simulink model "SF105A_MotCurrRegVltgLimr"  (R2013b)
settings: Solver=FixedStepDiscrete  SolverMode=SingleTasking  StartTime=0.0  StopTime=1  FixedStep=0.00025  RelTol=1e-3
undefined symbols (not defined in the file): ARCHGLBPRM_2OVERSQRT3_ULS_F32, ARCHGLBPRM_2PI_ULS_F32, BRDGVLTGHILIM_VOLT_F32, ELECGLBPRM_PWMPERDNOMX2_SEC_F32, F32TOU16OVR2PI_ULS_F32, MotCurrRegCfgCurrLoopSecOrderTrfFctEna, MotCurrRegCfgMotRVirtDax, MotCurrRegCfgMotRVirtQax, MotCurrRegVltgLimrCurrLoaScarSlewRate, MotCurrRegVltgLimrDaxAntiWdupCoeff, MotCurrRegVltgLimrDualEcuLoaScarSlewRate, MotCurrRegVltgLimrIvtrLoaScarSlewRate, MotCurrRegVltgLimrMotCurrPredEna, MotCurrRegVltgLimrMotCurrPredTi, MotCurrRegVltgLimrMotCurrQaxRefMdfnRplEna, MotCurrRegVltgLimrMotVltgBrdgFilEna, MotCurrRegVltgLimrMotVltgDaxIntglHiLim, MotCurrRegVltgLimrMotVltgDaxIntglLoLim, MotCurrRegVltgLimrMotVltgQaxFfFilEna, MotCurrRegVltgLimrMotVltgQaxIntglHiLim, MotCurrRegVltgLimrMotVltgQaxIntglLoLim, MotCurrRegVltgLimrQaxAntiWdupCoeff, MotCurrRegVltgLimrQaxAntiWdupScagDi, MotRefMdlFbCtrlDi, MotRefMdlIvtrDeadTiBrdgVltgSca, SysSt1, ZERO_VOLT_F32
libraries: NxtrLim x15, Fil x4, simulink x3, NxtrMax x2, NxtrMin x2
(part 3 of 5)

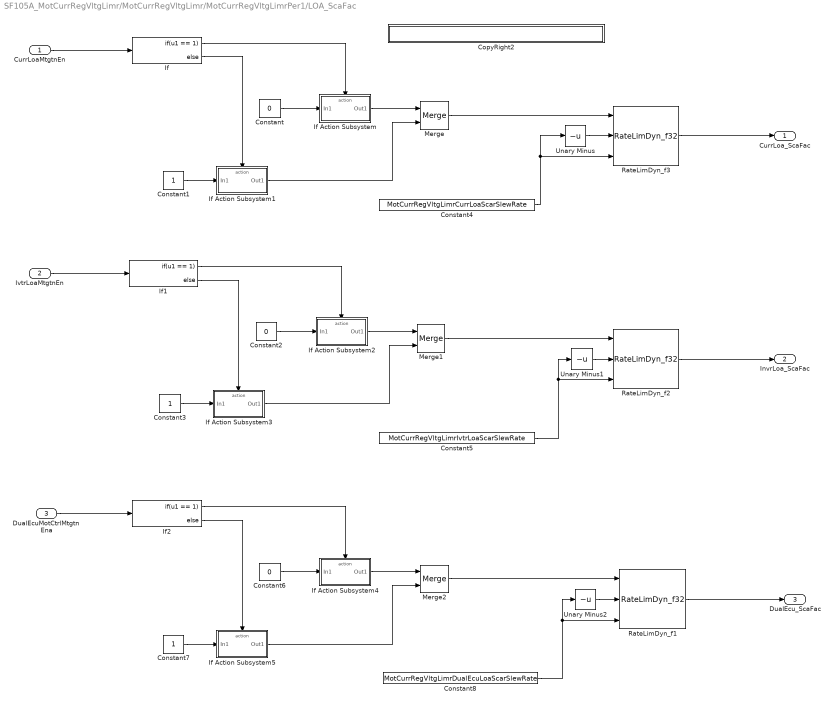
== system SF105A_MotCurrRegVltgLimr/MotCurrRegVltgLimr/MotCurrRegVltgLimrPer1/LOA_ScaFac ==
  CurrLoaMtgtnEn : Inport  RequirementInfo={'linktype_rmi_doors' '0000bb44 (/E-STEER Core/SubSystem Specifications/Application Functions/SF99/SF105A Current Regulator and Voltage Limiter)' '#SF105A_102' 'true' 'REQ: SF105A_102' '' } %GIDa_74016de8_2d3d_4e44_85d8_d4113689b030
  IvtrLoaMtgtnEn : Inport  RequirementInfo={'linktype_rmi_doors' '0000bb44 (/E-STEER Core/SubSystem Specifications/Application Functions/SF99/SF105A Current Regulator and Voltage Limiter)' '#SF105A_156' 'true' 'REQ: SF105A_156' '' } %GIDa_6f58899e_8eab_433e_baee_2993c9bd34be  Port=2
  DualEcuMotCtrlMtgtnEna : Inport  RequirementInfo={'linktype_rmi_doors' '0000bb44 (/E-STEER Core/SubSystem Specifications/Application Functions/SF99/SF105A Current Regulator and Voltage Limiter)' '#SF105A_156' 'true' 'REQ: SF105A_156' '' ; 'linktype_rmi_doors' '0000bb44 (/E-STEER Core/SubSystem Specifications/Application Functions/SF99/SF105A Current Regulator and Voltage Limiter)' '#SF105A_214' 'true' 'REQ: SF105A_214' '' } %GIDa_736db6b8_8a98_4c01_a4db_8969b61e8301  Port=3
  Constant : Constant  RequirementInfo={'linktype_rmi_doors' '0000bb44 (/E-STEER Core/SubSystem Specifications/Application Functions/SF99/SF105A Current Regulator and Voltage Limiter)' '#SF105A_102' 'true' 'REQ: SF105A_102' '' } %GIDa_9e5edeaa_9753_4523_84fc_d0edb0466ebb  Value=0  OutDataTypeStr=single
  Constant1 : Constant  RequirementInfo={'linktype_rmi_doors' '0000bb44 (/E-STEER Core/SubSystem Specifications/Application Functions/SF99/SF105A Current Regulator and Voltage Limiter)' '#SF105A_102' 'true' 'REQ: SF105A_102' '' } %GIDa_414e47fe_925f_4ace_960c_c6b1b25b4ef2  OutDataTypeStr=single
  Constant2 : Constant  RequirementInfo={'linktype_rmi_doors' '0000bb44 (/E-STEER Core/SubSystem Specifications/Application Functions/SF99/SF105A Current Regulator and Voltage Limiter)' '#SF105A_156' 'true' 'REQ: SF105A_156' '' } %GIDa_1b7b7f87_2781_4c0b_92e7_3da3ba5adda7  Value=0  OutDataTypeStr=single
  Constant3 : Constant  RequirementInfo={'linktype_rmi_doors' '0000bb44 (/E-STEER Core/SubSystem Specifications/Application Functions/SF99/SF105A Current Regulator and Voltage Limiter)' '#SF105A_156' 'true' 'REQ: SF105A_156' '' } %GIDa_009e418e_db5b_41d9_ae78_f46b7f47c2f9  OutDataTypeStr=single
  Constant4 : Constant  RequirementInfo={'linktype_rmi_doors' '0000bb44 (/E-STEER Core/SubSystem Specifications/Application Functions/SF99/SF105A Current Regulator and Voltage Limiter)' '#SF105A_101' 'true' 'REQ: SF105A_101' '' } %GIDa_4127ceec_6765_4e92_b839_f1bde89d8c0b  Value=MotCurrRegVltgLimrCurrLoaScarSlewRate
  Constant5 : Constant  RequirementInfo={'linktype_rmi_doors' '0000bb44 (/E-STEER Core/SubSystem Specifications/Application Functions/SF99/SF105A Current Regulator and Voltage Limiter)' '#SF105A_158' 'true' 'REQ: SF105A_158' '' } %GIDa_d375279a_c0b4_445f_88b4_097dc89d2371  Value=MotCurrRegVltgLimrIvtrLoaScarSlewRate
  Constant6 : Constant  RequirementInfo={'linktype_rmi_doors' '0000bb44 (/E-STEER Core/SubSystem Specifications/Application Functions/SF99/SF105A Current Regulator and Voltage Limiter)' '#SF105A_156' 'true' 'REQ: SF105A_156' '' ; 'linktype_rmi_doors' '0000bb44 (/E-STEER Core/SubSystem Specifications/Application Functions/SF99/SF105A Current Regulator and Voltage Limiter)' '#SF105A_214' 'true' 'REQ: SF105A_214' '' } %GIDa_1132c686_87fe_415f_a0bc_4e5d655024ab  Value=0  OutDataTypeStr=single
  Constant7 : Constant  RequirementInfo={'linktype_rmi_doors' '0000bb44 (/E-STEER Core/SubSystem Specifications/Application Functions/SF99/SF105A Current Regulator and Voltage Limiter)' '#SF105A_156' 'true' 'REQ: SF105A_156' '' ; 'linktype_rmi_doors' '0000bb44 (/E-STEER Core/SubSystem Specifications/Application Functions/SF99/SF105A Current Regulator and Voltage Limiter)' '#SF105A_214' 'true' 'REQ: SF105A_214' '' } %GIDa_7ef12da6_ad43_483e_a835_c5dd150fe6fe  OutDataTypeStr=single
  Constant8 : Constant  RequirementInfo={'linktype_rmi_doors' '0000bb44 (/E-STEER Core/SubSystem Specifications/Application Functions/SF99/SF105A Current Regulator and Voltage Limiter)' '#SF105A_213' 'true' 'REQ: SF105A_213' '' } %GIDa_fc42a242_7564_4710_9c19_eef5c8ae2cee  Value=MotCurrRegVltgLimrDualEcuLoaScarSlewRate
  CopyRight2 : Subsystem  Description=|  mask(Copyright Information){none=on}
      | Copyright info block.                                               
      |                                                                     
      | Place copyright information at the top of every subsystem in design.
      mask prompts: none "No parameters"
      mask help: Place copyright information at the top of every subsystem in design.
      mask Display:
      | NxtrConf = 'Nexteer Confidential';
      | 
      | sys = bdroot; %handle for the current model ("system")
      | first = get_param(sys,'Created');
      | if(isempty(first))
      |     first = datestr(now,'yyyy');
      | else
      |     first = first(end-3:end);  %year is last four digits
      | end
      | 
      | last = get_param(sys,'LastModifiedDate');
      | if isempty(last)
      |     last = datestr(now,'yyyy');
      | else
      |     last = last(end-3:end);
      | end
      | 
      | if strcmp(first,last)
      |     fprintf('%s -- Copyright %s Nexteer',NxtrConf,first)
      | else
      |     fprintf('%s -- %s%s- %s Nexteer',NxtrConf,char(169),first,last)
      | end
  If : If  RequirementInfo={'linktype_rmi_doors' '0000bb44 (/E-STEER Core/SubSystem Specifications/Application Functions/SF99/SF105A Current Regulator and Voltage Limiter)' '#SF105A_102' 'true' 'REQ: SF105A_102' '' } %GIDa_3a91bae6_7fe9_4df3_8189_f002690391f2  IfExpression=u1 == 1
  If Action Subsystem : Subsystem  RequirementInfo={'linktype_rmi_doors' '0000bb44 (/E-STEER Core/SubSystem Specifications/Application Functions/SF99/SF105A Current Regulator and Voltage Limiter)' '#SF105A_102' 'true' 'REQ: SF105A_102' '' } %GIDa_4746905c_4450_4de8_aeb6_d31492493c35  TreatAsAtomicUnit=on
  If Action Subsystem1 : Subsystem  RequirementInfo={'linktype_rmi_doors' '0000bb44 (/E-STEER Core/SubSystem Specifications/Application Functions/SF99/SF105A Current Regulator and Voltage Limiter)' '#SF105A_102' 'true' 'REQ: SF105A_102' '' } %GIDa_3824dd5c_a3c5_4e02_bf52_4a1d9300439b  TreatAsAtomicUnit=on
  If Action Subsystem2 : Subsystem  RequirementInfo={'linktype_rmi_doors' '0000bb44 (/E-STEER Core/SubSystem Specifications/Application Functions/SF99/SF105A Current Regulator and Voltage Limiter)' '#SF105A_156' 'true' 'REQ: SF105A_156' '' } %GIDa_1af216f2_cb25_4b77_bb8c_abc2dc18253e  TreatAsAtomicUnit=on
  If Action Subsystem3 : Subsystem  RequirementInfo={'linktype_rmi_doors' '0000bb44 (/E-STEER Core/SubSystem Specifications/Application Functions/SF99/SF105A Current Regulator and Voltage Limiter)' '#SF105A_156' 'true' 'REQ: SF105A_156' '' } %GIDa_f1b7b46f_b59a_420d_a525_ef233d17b094  TreatAsAtomicUnit=on
  If Action Subsystem4 : Subsystem  RequirementInfo={'linktype_rmi_doors' '0000bb44 (/E-STEER Core/SubSystem Specifications/Application Functions/SF99/SF105A Current Regulator and Voltage Limiter)' '#SF105A_156' 'true' 'REQ: SF105A_156' '' ; 'linktype_rmi_doors' '0000bb44 (/E-STEER Core/SubSystem Specifications/Application Functions/SF99/SF105A Current Regulator and Voltage Limiter)' '#SF105A_214' 'true' 'REQ: SF105A_214' '' } %GIDa_6d2e553f_9dcf_4646_b57e_342b22099bc6  TreatAsAtomicUnit=on
  If Action Subsystem5 : Subsystem  RequirementInfo={'linktype_rmi_doors' '0000bb44 (/E-STEER Core/SubSystem Specifications/Application Functions/SF99/SF105A Current Regulator and Voltage Limiter)' '#SF105A_156' 'true' 'REQ: SF105A_156' '' ; 'linktype_rmi_doors' '0000bb44 (/E-STEER Core/SubSystem Specifications/Application Functions/SF99/SF105A Current Regulator and Voltage Limiter)' '#SF105A_214' 'true' 'REQ: SF105A_214' '' } %GIDa_45a5a307_dfa1_464a_845e_5937a4578355  TreatAsAtomicUnit=on
  If1 : If  RequirementInfo={'linktype_rmi_doors' '0000bb44 (/E-STEER Core/SubSystem Specifications/Application Functions/SF99/SF105A Current Regulator and Voltage Limiter)' '#SF105A_156' 'true' 'REQ: SF105A_156' '' } %GIDa_08038fbf_a660_4706_ace0_908cef9a7a3c  IfExpression=u1 == 1
  If2 : If  RequirementInfo={'linktype_rmi_doors' '0000bb44 (/E-STEER Core/SubSystem Specifications/Application Functions/SF99/SF105A Current Regulator and Voltage Limiter)' '#SF105A_156' 'true' 'REQ: SF105A_156' '' ; 'linktype_rmi_doors' '0000bb44 (/E-STEER Core/SubSystem Specifications/Application Functions/SF99/SF105A Current Regulator and Voltage Limiter)' '#SF105A_214' 'true' 'REQ: SF105A_214' '' } %GIDa_d47c7b75_0445_4629_a8f6_7d3cc89f6b1e  IfExpression=u1 == 1
  Merge : Merge  RequirementInfo={'linktype_rmi_doors' '0000bb44 (/E-STEER Core/SubSystem Specifications/Application Functions/SF99/SF105A Current Regulator and Voltage Limiter)' '#SF105A_102' 'true' 'REQ: SF105A_102' '' } %GIDa_02e5c2a5_d864_4ef7_8f58_89b7f0e83ac4
  Merge1 : Merge  RequirementInfo={'linktype_rmi_doors' '0000bb44 (/E-STEER Core/SubSystem Specifications/Application Functions/SF99/SF105A Current Regulator and Voltage Limiter)' '#SF105A_156' 'true' 'REQ: SF105A_156' '' } %GIDa_1411ac7b_0602_4079_91ff_3bf75b7f8933
  Merge2 : Merge  RequirementInfo={'linktype_rmi_doors' '0000bb44 (/E-STEER Core/SubSystem Specifications/Application Functions/SF99/SF105A Current Regulator and Voltage Limiter)' '#SF105A_156' 'true' 'REQ: SF105A_156' '' ; 'linktype_rmi_doors' '0000bb44 (/E-STEER Core/SubSystem Specifications/Application Functions/SF99/SF105A Current Regulator and Voltage Limiter)' '#SF105A_214' 'true' 'REQ: SF105A_214' '' } %GIDa_b21e043f_9e48_4dac_a088_0ae5e3077f20
  RateLimDyn_f1 : NxtrLim/RateLimDyn_f32  RequirementInfo={'linktype_rmi_doors' '0000bb44 (/E-STEER Core/SubSystem Specifications/Application Functions/SF99/SF105A Current Regulator and Voltage Limiter)' '#SF105A_215' 'true' 'REQ: SF105A_215' '' } %GIDa_febcb8d3_d490_462d_9585_cc90d4e1d855  StVar=DualEcuLoaScarPrev  Ts=ELECGLBPRM_PWMPERDNOMX2_SEC_F32
      settings: AttributesFormatString=StVar: %<StVar>
  RateLimDyn_f2 : NxtrLim/RateLimDyn_f32  StVar=IvtrLoaScarPrev  Ts=ELECGLBPRM_PWMPERDNOMX2_SEC_F32
      settings: AttributesFormatString=StVar: %<StVar>
  RateLimDyn_f3 : NxtrLim/RateLimDyn_f32  StVar=CurrLoaScarPrev  Ts=ELECGLBPRM_PWMPERDNOMX2_SEC_F32
      settings: AttributesFormatString=StVar: %<StVar>
  Unary Minus : UnaryMinus  RequirementInfo={'linktype_rmi_doors' '0000bb44 (/E-STEER Core/SubSystem Specifications/Application Functions/SF99/SF105A Current Regulator and Voltage Limiter)' '#SF105A_101' 'true' 'REQ: SF105A_101' '' } %GIDa_2742d1db_4c29_4c43_bc00_21ac76a60273
  Unary Minus1 : UnaryMinus  RequirementInfo={'linktype_rmi_doors' '0000bb44 (/E-STEER Core/SubSystem Specifications/Application Functions/SF99/SF105A Current Regulator and Voltage Limiter)' '#SF105A_158' 'true' 'REQ: SF105A_158' '' } %GIDa_35918956_e63f_4f48_ad3b_713daa2d1a68
  Unary Minus2 : UnaryMinus  RequirementInfo={'linktype_rmi_doors' '0000bb44 (/E-STEER Core/SubSystem Specifications/Application Functions/SF99/SF105A Current Regulator and Voltage Limiter)' '#SF105A_158' 'true' 'REQ: SF105A_158' '' } %GIDa_c3ad0f7f_3bfe_4cdc_ba65_f783df0f12a2
  CurrLoa_ScaFac : Outport  RequirementInfo={'linktype_rmi_doors' '0000bb44 (/E-STEER Core/SubSystem Specifications/Application Functions/SF99/SF105A Current Regulator and Voltage Limiter)' '#SF105A_102' 'true' 'REQ: SF105A_102' '' } %GIDa_45fecacb_2175_43de_a689_6a1c7683416a
  InvrLoa_ScaFac : Outport  RequirementInfo={'linktype_rmi_doors' '0000bb44 (/E-STEER Core/SubSystem Specifications/Application Functions/SF99/SF105A Current Regulator and Voltage Limiter)' '#SF105A_156' 'true' 'REQ: SF105A_156' '' } %GIDa_392678cc_9a17_4a2c_ba15_6492b437acac  Port=2
  DualEcu_ScaFac : Outport  RequirementInfo={'linktype_rmi_doors' '0000bb44 (/E-STEER Core/SubSystem Specifications/Application Functions/SF99/SF105A Current Regulator and Voltage Limiter)' '#SF105A_156' 'true' 'REQ: SF105A_156' '' } %GIDa_aaab24fd_64b0_48fa_9ed0_c4d4e741348c  Port=3
  wires:
  RateLimDyn_f3/1 -> CurrLoa_ScaFac/1
  RateLimDyn_f2/1 -> InvrLoa_ScaFac/1
  CurrLoaMtgtnEn/1 -> If/1
  If/1 -> If Action Subsystem/Action
  If/2 -> If Action Subsystem1/Action
  If Action Subsystem/1(Out1) -> Merge/1
  If Action Subsystem1/1(Out1) -> Merge/2
  Merge/1 -> RateLimDyn_f3/1
  Constant/1 -> If Action Subsystem/1(In1)
  Constant1/1 -> If Action Subsystem1/1(In1)
  If1/1 -> If Action Subsystem2/Action
  If1/2 -> If Action Subsystem3/Action
  If Action Subsystem2/1(Out1) -> Merge1/1
  If Action Subsystem3/1(Out1) -> Merge1/2
  Constant2/1 -> If Action Subsystem2/1(In1)
  Constant3/1 -> If Action Subsystem3/1(In1)
  Merge1/1 -> RateLimDyn_f2/1
  IvtrLoaMtgtnEn/1 -> If1/1
  Unary Minus/1 -> RateLimDyn_f3/2
  Constant4/1 -> RateLimDyn_f3/3, Unary Minus/1
  Constant5/1 -> RateLimDyn_f2/3, Unary Minus1/1
  Unary Minus1/1 -> RateLimDyn_f2/2
  RateLimDyn_f1/1 -> DualEcu_ScaFac/1
  If2/1 -> If Action Subsystem4/Action
  If2/2 -> If Action Subsystem5/Action
  If Action Subsystem4/1(Out1) -> Merge2/1
  If Action Subsystem5/1(Out1) -> Merge2/2
  Constant6/1 -> If Action Subsystem4/1(In1)
  Constant7/1 -> If Action Subsystem5/1(In1)
  Merge2/1 -> RateLimDyn_f1/1
  DualEcuMotCtrlMtgtnEna/1 -> If2/1
  Constant8/1 -> RateLimDyn_f1/3, Unary Minus2/1
  Unary Minus2/1 -> RateLimDyn_f1/2

== system SF105A_MotCurrRegVltgLimr/MotCurrRegVltgLimr/MotCurrRegVltgLimrPer1/MotCurr_ErrCalc_Dax ==
  MotCurr_DaxCmd : Inport  RequirementInfo={'linktype_rmi_doors' '0000bb44 (/E-STEER Core/SubSystem Specifications/Application Functions/SF99/SF105A Current Regulator and Voltage Limiter)' '#SF105A_79' 'true' 'REQ: SF105A_79' '' } %GIDa_9f860954_e875_4c8d_8e1d_5693f49ff45b
  MotCurr_DaxCmd_Max : Inport  RequirementInfo={'linktype_rmi_doors' '0000bb44 (/E-STEER Core/SubSystem Specifications/Application Functions/SF99/SF105A Current Regulator and Voltage Limiter)' '#SF105A_79' 'true' 'REQ: SF105A_79' '' } %GIDa_059e93a2_947a_47bb_8dd6_2243dd2f4f72  Port=2
  MotCurrModif_Dax : Inport  RequirementInfo={'linktype_rmi_doors' '0000bb44 (/E-STEER Core/SubSystem Specifications/Application Functions/SF99/SF105A Current Regulator and Voltage Limiter)' '#SF105A_80' 'true' 'REQ: SF105A_80' '' } %GIDa_0a5f56fa_a877_4df4_9019_19b65ccf742b  Port=3
  AntiWdup_CmdScag_Dax : Inport  RequirementInfo={'linktype_rmi_doors' '0000bb44 (/E-STEER Core/SubSystem Specifications/Application Functions/SF99/SF105A Current Regulator and Voltage Limiter)' '#SF105A_79' 'true' 'REQ: SF105A_79' '' } %GIDa_16448b7e_ab4b_4b1d_9cde_07b89661d2d9  Port=4
  Add : Sum  RequirementInfo={'linktype_rmi_doors' '0000bb44 (/E-STEER Core/SubSystem Specifications/Application Functions/SF99/SF105A Current Regulator and Voltage Limiter)' '#SF105A_79' 'true' 'REQ: SF105A_79' '' } %GIDa_39dd1027_d310_4f71_96a2_2a266e8bfe38  Inputs=-+
  Add1 : Sum  RequirementInfo={'linktype_rmi_doors' '0000bb44 (/E-STEER Core/SubSystem Specifications/Application Functions/SF99/SF105A Current Regulator and Voltage Limiter)' '#SF105A_79' 'true' 'REQ: SF105A_79' '' ; 'linktype_rmi_doors' '0000bb44 (/E-STEER Core/SubSystem Specifications/Application Functions/SF99/SF105A Current Regulator and Voltage Limiter)' '#SF105A_80' 'true' 'REQ: SF105A_80' '' } %GIDa_29048c9a_b932_4a00_8976_f9e9609904a4
  Add2 : Sum  RequirementInfo={'linktype_rmi_doors' '0000bb44 (/E-STEER Core/SubSystem Specifications/Application Functions/SF99/SF105A Current Regulator and Voltage Limiter)' '#SF105A_80' 'true' 'REQ: SF105A_80' '' } %GIDa_390b17ed_9d59_44c9_82bb_54ff4b90a4f8  Inputs=+-
  Constant : Constant  RequirementInfo={'linktype_rmi_doors' '0000bb44 (/E-STEER Core/SubSystem Specifications/Application Functions/SF99/SF105A Current Regulator and Voltage Limiter)' '#SF105A_79' 'true' 'REQ: SF105A_79' '' } %GIDa_71ff8474_cc08_4c6f_98c7_9495352e7f22  OutDataTypeStr=single
  CopyRight2 : Subsystem  Description=|  mask(Copyright Information){none=on}
      | Copyright info block.                                               
      |                                                                     
      | Place copyright information at the top of every subsystem in design.
      mask prompts: none "No parameters"
      mask help: Place copyright information at the top of every subsystem in design.
      mask Display:
      | NxtrConf = 'Nexteer Confidential';
      | 
      | sys = bdroot; %handle for the current model ("system")
      | first = get_param(sys,'Created');
      | if(isempty(first))
      |     first = datestr(now,'yyyy');
      | else
      |     first = first(end-3:end);  %year is last four digits
      | end
      | 
      | last = get_param(sys,'LastModifiedDate');
      | if isempty(last)
      |     last = datestr(now,'yyyy');
      | else
      |     last = last(end-3:end);
      | end
      | 
      | if strcmp(first,last)
      |     fprintf('%s -- Copyright %s Nexteer',NxtrConf,first)
      | else
      |     fprintf('%s -- %s%s- %s Nexteer',NxtrConf,char(169),first,last)
      | end
  Data Store Write : DataStoreWrite  DataStoreName=dMotCurrRegVltgLimrMotCurrCmdScaDax
  Data Store Write1 : DataStoreWrite  DataStoreName=dMotCurrRegVltgLimrMotCurrCmdErrDax
  LimStat_f32 : NxtrLim/LimStat_f32  RequirementInfo={'linktype_rmi_doors' '0000bb44 (/E-STEER Core/SubSystem Specifications/Application Functions/SF99/SF105A Current Regulator and Voltage Limiter)' '#SF105A_194' 'true' 'REQ: SF105A_194' '' } %GIDa_41824742_1c4e_4aae_9c40_6d1680dffacc  LoLim=0  HiLim=MOTCURRHILIM_AMPR_F32
      settings: AttributesFormatString=|
      | Low Limit: %<LoLim>
      | High Limit:%<HiLim>
  Product : Product  RequirementInfo={'linktype_rmi_doors' '0000bb44 (/E-STEER Core/SubSystem Specifications/Application Functions/SF99/SF105A Current Regulator and Voltage Limiter)' '#SF105A_79' 'true' 'REQ: SF105A_79' '' } %GIDa_865b35e4_9b9d_4019_bb82_f747255cb73b
  Product1 : Product  RequirementInfo={'linktype_rmi_doors' '0000bb44 (/E-STEER Core/SubSystem Specifications/Application Functions/SF99/SF105A Current Regulator and Voltage Limiter)' '#SF105A_79' 'true' 'REQ: SF105A_79' '' } %GIDa_d60d7378_f447_4ef8_b073_e1658ac34c86
  CmdErr_Dax : Outport  RequirementInfo={'linktype_rmi_doors' '0000bb44 (/E-STEER Core/SubSystem Specifications/Application Functions/SF99/SF105A Current Regulator and Voltage Limiter)' '#SF105A_80' 'true' 'REQ: SF105A_80' '' } %GIDa_fb394d4d_5f75_43b4_b8c6_8763df3a229d
  wires:
  MotCurr_DaxCmd/1 -> Product/1
  AntiWdup_CmdScag_Dax/1 -> Product/2, Add/1
  Constant/1 -> Add/2
  Add/1 -> Product1/1
  MotCurr_DaxCmd_Max/1 -> Product1/2
  Product1/1 -> Add1/2
  Product/1 -> Add1/1
  Add1/1 -> LimStat_f32/1
  Add2/1 -> Data Store Write1/1, CmdErr_Dax/1
  MotCurrModif_Dax/1 -> Add2/2
  LimStat_f32/1 -> Add2/1, Data Store Write/1

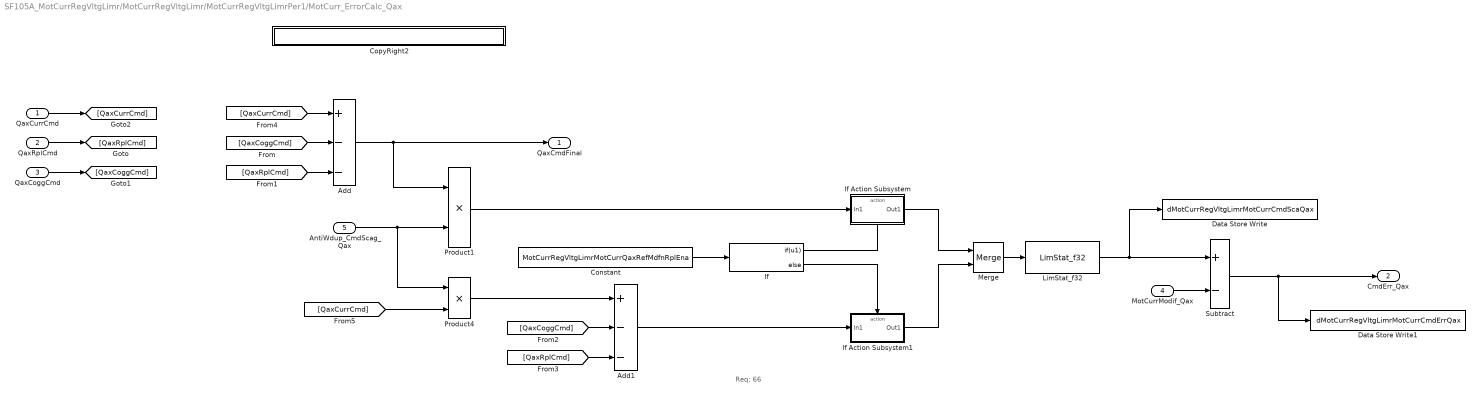
== system SF105A_MotCurrRegVltgLimr/MotCurrRegVltgLimr/MotCurrRegVltgLimrPer1/MotCurr_ErrorCalc_Qax ==
  note: Req: 66
  QaxCurrCmd : Inport
  QaxRplCmd : Inport  Port=2
  QaxCoggCmd : Inport  Port=3
  MotCurrModif_Qax : Inport  RequirementInfo={'linktype_rmi_doors' '0000bb44 (/E-STEER Core/SubSystem Specifications/Application Functions/SF99/SF105A Current Regulator and Voltage Limiter)' '#SF105A_68' 'true' 'REQ: SF105A_68' '' } %GIDa_7ddb042c_949f_40bd_a5a0_caaccdad8aec  Port=4
  AntiWdup_CmdScag_Qax : Inport  RequirementInfo={'linktype_rmi_doors' '0000bb44 (/E-STEER Core/SubSystem Specifications/Application Functions/SF99/SF105A Current Regulator and Voltage Limiter)' '#SF105A_66' 'true' 'REQ: SF105A_66' '' } %GIDa_f11ef98d_60e0_4a29_bcf5_371694c4b8ce  Port=5
  Add : Sum  RequirementInfo={'linktype_rmi_doors' '0000bb44 (/E-STEER Core/SubSystem Specifications/Application Functions/SF99/SF105A Current Regulator and Voltage Limiter)' '#SF105A_67' 'true' 'REQ: SF105A_67' '' } %GIDa_824a2f17_525f_4037_bf25_6f84ed62cd1c  Inputs=+--
  Add1 : Sum  RequirementInfo={'linktype_rmi_doors' '0000bb44 (/E-STEER Core/SubSystem Specifications/Application Functions/SF99/SF105A Current Regulator and Voltage Limiter)' '#SF105A_67' 'true' 'REQ: SF105A_67' '' ; 'linktype_rmi_doors' '0000bb44 (/E-STEER Core/SubSystem Specifications/Application Functions/SF99/SF105A Current Regulator and Voltage Limiter)' '#SF105A_68' 'true' 'REQ: SF105A_68' '' ; 'linktype_rmi_doors' '0000bb44 (/E-STEER Core/SubSystem Specifications/Application Functions/SF99/SF105A Current Regulator and Voltage Limiter)' '#SF105A_66' 'true' 'REQ: SF105A_66' '' } %GIDa_68034fa4_dd2b_4432_96f4_ee6556315ecf  Inputs=+--
  Constant : Constant  RequirementInfo={'linktype_rmi_doors' '0000bb44 (/E-STEER Core/SubSystem Specifications/Application Functions/SF99/SF105A Current Regulator and Voltage Limiter)' '#SF105A_66' 'true' 'REQ: SF105A_66' '' } %GIDa_9ec7087e_f41f_4423_86a7_6e625803caeb  Value=MotCurrRegVltgLimrMotCurrQaxRefMdfnRplEna
  CopyRight2 : Subsystem  Description=|  mask(Copyright Information){none=on}
      | Copyright info block.                                               
      |                                                                     
      | Place copyright information at the top of every subsystem in design.
      mask prompts: none "No parameters"
      mask help: Place copyright information at the top of every subsystem in design.
      mask Display:
      | NxtrConf = 'Nexteer Confidential';
      | 
      | sys = bdroot; %handle for the current model ("system")
      | first = get_param(sys,'Created');
      | if(isempty(first))
      |     first = datestr(now,'yyyy');
      | else
      |     first = first(end-3:end);  %year is last four digits
      | end
      | 
      | last = get_param(sys,'LastModifiedDate');
      | if isempty(last)
      |     last = datestr(now,'yyyy');
      | else
      |     last = last(end-3:end);
      | end
      | 
      | if strcmp(first,last)
      |     fprintf('%s -- Copyright %s Nexteer',NxtrConf,first)
      | else
      |     fprintf('%s -- %s%s- %s Nexteer',NxtrConf,char(169),first,last)
      | end
  Data Store Write : DataStoreWrite  DataStoreName=dMotCurrRegVltgLimrMotCurrCmdScaQax
  Data Store Write1 : DataStoreWrite  DataStoreName=dMotCurrRegVltgLimrMotCurrCmdErrQax
  If : If  RequirementInfo={'linktype_rmi_doors' '0000bb44 (/E-STEER Core/SubSystem Specifications/Application Functions/SF99/SF105A Current Regulator and Voltage Limiter)' '#SF105A_66' 'true' 'REQ: SF105A_66' '' } %GIDa_3422f6ba_ed31_4d28_a209_ee709dd11907  IfExpression=u1
  If Action Subsystem : Subsystem  RequirementInfo={'linktype_rmi_doors' '0000bb44 (/E-STEER Core/SubSystem Specifications/Application Functions/SF99/SF105A Current Regulator and Voltage Limiter)' '#SF105A_66' 'true' 'REQ: SF105A_66' '' } %GIDa_cff3645e_70eb_479a_8cd2_a8659d70b1bb  TreatAsAtomicUnit=on
  If Action Subsystem1 : Subsystem  RequirementInfo={'linktype_rmi_doors' '0000bb44 (/E-STEER Core/SubSystem Specifications/Application Functions/SF99/SF105A Current Regulator and Voltage Limiter)' '#SF105A_66' 'true' 'REQ: SF105A_66' '' } %GIDa_5c53fa27_9bd9_46be_8574_f721519fc2a6  TreatAsAtomicUnit=on
  LimStat_f32 : NxtrLim/LimStat_f32  RequirementInfo={'linktype_rmi_doors' '0000bb44 (/E-STEER Core/SubSystem Specifications/Application Functions/SF99/SF105A Current Regulator and Voltage Limiter)' '#SF105A_192' 'true' 'REQ: SF105A_192' '' } %GIDa_31cf29ce_c2ae_4e26_a267_244a0aa9250f  LoLim=MOTCURRLOLIM_AMPR_F32  HiLim=MOTCURRHILIM_AMPR_F32
      settings: AttributesFormatString=|
      | Low Limit: %<LoLim>
      | High Limit:%<HiLim>
  Merge : Merge  RequirementInfo={'linktype_rmi_doors' '0000bb44 (/E-STEER Core/SubSystem Specifications/Application Functions/SF99/SF105A Current Regulator and Voltage Limiter)' '#SF105A_66' 'true' 'REQ: SF105A_66' '' } %GIDa_0142320b_7588_4c2a_92e0_9d1571f759a1
  Product1 : Product  RequirementInfo={'linktype_rmi_doors' '0000bb44 (/E-STEER Core/SubSystem Specifications/Application Functions/SF99/SF105A Current Regulator and Voltage Limiter)' '#SF105A_66' 'true' 'REQ: SF105A_66' '' } %GIDa_00046f93_3b3c_43ee_b28c_8f0dba5d6301
  Product4 : Product  RequirementInfo={'linktype_rmi_doors' '0000bb44 (/E-STEER Core/SubSystem Specifications/Application Functions/SF99/SF105A Current Regulator and Voltage Limiter)' '#SF105A_66' 'true' 'REQ: SF105A_66' '' ; 'linktype_rmi_doors' '0000bb44 (/E-STEER Core/SubSystem Specifications/Application Functions/SF99/SF105A Current Regulator and Voltage Limiter)' '#SF105A_67' 'true' 'REQ: SF105A_67' '' ; 'linktype_rmi_doors' '0000bb44 (/E-STEER Core/SubSystem Specifications/Application Functions/SF99/SF105A Current Regulator and Voltage Limiter)' '#SF105A_66' 'true' 'REQ: SF105A_66' '' } %GIDa_5eda651c_d9cf_4592_83a1_ad2c6ced6304
  Subtract : Sum  RequirementInfo={'linktype_rmi_doors' '0000bb44 (/E-STEER Core/SubSystem Specifications/Application Functions/SF99/SF105A Current Regulator and Voltage Limiter)' '#SF105A_68' 'true' 'REQ: SF105A_68' '' } %GIDa_847c6db2_b488_4579_a9b0_6b38d1c11d10  Inputs=+-
  QaxCmdFinal : Outport
  CmdErr_Qax : Outport  RequirementInfo={'linktype_rmi_doors' '0000bb44 (/E-STEER Core/SubSystem Specifications/Application Functions/SF99/SF105A Current Regulator and Voltage Limiter)' '#SF105A_68' 'true' 'REQ: SF105A_68' '' } %GIDa_89496b6d_771a_4c11_b3f5_27b7e28477ad  Port=2
  wires:
  [QaxCurrCmd] -> Product4/2
  MotCurrModif_Qax/1 -> Subtract/2
  Subtract/1 -> Data Store Write1/1, CmdErr_Qax/1
  Product4/1 -> Add1/1
  Add1/1 -> If Action Subsystem1/1(In1)
  QaxRplCmd/1 -> [QaxRplCmd]
  QaxCoggCmd/1 -> [QaxCoggCmd]
  [QaxCoggCmd] -> Add/2
  [QaxRplCmd] -> Add/3
  [QaxCoggCmd] -> Add1/2
  [QaxRplCmd] -> Add1/3
  QaxCurrCmd/1 -> [QaxCurrCmd]
  [QaxCurrCmd] -> Add/1
  AntiWdup_CmdScag_Qax/1 -> Product4/1, Product1/2
  Add/1 -> Product1/1, QaxCmdFinal/1
  Product1/1 -> If Action Subsystem/1(In1)
  Constant/1 -> If/1
  If/1 -> If Action Subsystem/Action
  If/2 -> If Action Subsystem1/Action
  If Action Subsystem1/1(Out1) -> Merge/2
  If Action Subsystem/1(Out1) -> Merge/1
  Merge/1 -> LimStat_f32/1
  LimStat_f32/1 -> Data Store Write/1, Subtract/1

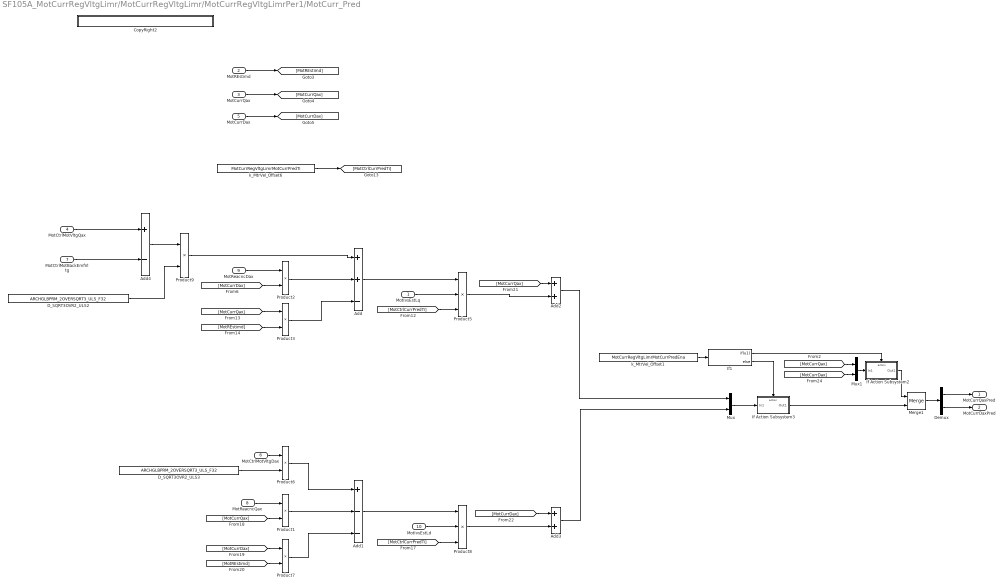
== system SF105A_MotCurrRegVltgLimr/MotCurrRegVltgLimr/MotCurrRegVltgLimrPer1/MotCurr_Pred ==
  MotIvsEstLq : Inport  RequirementInfo={'linktype_rmi_doors' '0000bb44 (/E-STEER Core/SubSystem Specifications/Application Functions/SF99/SF105A Current Regulator and Voltage Limiter)' '#SF105A_212' 'true' 'REQ: SF105A_212' '' } %GIDa_3aeb3707_45ce_487a_b4ed_ddb2c28398c2
  MotREstimd : Inport  Port=2
  MotCurrQax : Inport  Port=3
  MotCtrlMotVltgQax : Inport  RequirementInfo={'linktype_rmi_doors' '0000bb44 (/E-STEER Core/SubSystem Specifications/Application Functions/SF99/SF105A Current Regulator and Voltage Limiter)' '#SF105A_212' 'true' 'REQ: SF105A_212' '' } %GIDa_1ecf2394_21d0_40ef_b0e3_5db783a06b70  Port=4
  MotCurrDax : Inport  Port=5
  MotCtrlMotVltgDax : Inport  RequirementInfo={'linktype_rmi_doors' '0000bb44 (/E-STEER Core/SubSystem Specifications/Application Functions/SF99/SF105A Current Regulator and Voltage Limiter)' '#SF105A_212' 'true' 'REQ: SF105A_212' '' } %GIDa_5e37510e_3e03_4149_b438_6d1de96fc9bd  Port=6
  MotCtrlMotBackEmfVltg : Inport  RequirementInfo={'linktype_rmi_doors' '0000bb44 (/E-STEER Core/SubSystem Specifications/Application Functions/SF99/SF105A Current Regulator and Voltage Limiter)' '#SF105A_212' 'true' 'REQ: SF105A_212' '' } %GIDa_765cd72c_424b_447b_899f_bcea498ee91a  Port=7
  MotReacncQax : Inport  RequirementInfo={'linktype_rmi_doors' '0000bb44 (/E-STEER Core/SubSystem Specifications/Application Functions/SF99/SF105A Current Regulator and Voltage Limiter)' '#SF105A_212' 'true' 'REQ: SF105A_212' '' } %GIDa_bb9a6fa6_bb3a_4e91_a529_41e679c1d7ff  Port=8
  MotReacncDax : Inport  RequirementInfo={'linktype_rmi_doors' '0000bb44 (/E-STEER Core/SubSystem Specifications/Application Functions/SF99/SF105A Current Regulator and Voltage Limiter)' '#SF105A_212' 'true' 'REQ: SF105A_212' '' } %GIDa_28f35d53_2518_44d1_87e5_ea55ef80b988  Port=9
  MotIvsEstLd : Inport  RequirementInfo={'linktype_rmi_doors' '0000bb44 (/E-STEER Core/SubSystem Specifications/Application Functions/SF99/SF105A Current Regulator and Voltage Limiter)' '#SF105A_212' 'true' 'REQ: SF105A_212' '' } %GIDa_ff070b0f_2e16_4e29_b62f_6a4f9be963a3  Port=10
  Add : Sum  RequirementInfo={'linktype_rmi_doors' '0000bb44 (/E-STEER Core/SubSystem Specifications/Application Functions/SF99/SF105A Current Regulator and Voltage Limiter)' '#SF105A_212' 'true' 'REQ: SF105A_212' '' } %GIDa_ac1688c1_716b_4d53_ab90_d2b44201a94d  Inputs=++-
  Add1 : Sum  RequirementInfo={'linktype_rmi_doors' '0000bb44 (/E-STEER Core/SubSystem Specifications/Application Functions/SF99/SF105A Current Regulator and Voltage Limiter)' '#SF105A_212' 'true' 'REQ: SF105A_212' '' } %GIDa_2bda87c1_f458_4474_bec5_9fab776bf9d1  Inputs=+--
  Add2 : Sum  RequirementInfo={'linktype_rmi_doors' '0000bb44 (/E-STEER Core/SubSystem Specifications/Application Functions/SF99/SF105A Current Regulator and Voltage Limiter)' '#SF105A_212' 'true' 'REQ: SF105A_212' '' } %GIDa_1ee4b117_3144_4e79_9ffc_51afd2a704e2
  Add3 : Sum  RequirementInfo={'linktype_rmi_doors' '0000bb44 (/E-STEER Core/SubSystem Specifications/Application Functions/SF99/SF105A Current Regulator and Voltage Limiter)' '#SF105A_212' 'true' 'REQ: SF105A_212' '' } %GIDa_27e9bb07_36e4_445b_9822_5fd190a22332
  Add4 : Sum  RequirementInfo={'linktype_rmi_doors' '0000bb44 (/E-STEER Core/SubSystem Specifications/Application Functions/SF99/SF105A Current Regulator and Voltage Limiter)' '#SF105A_212' 'true' 'REQ: SF105A_212' '' } %GIDa_9b0a0a47_5e7d_4595_92d7_59c1ca4f205f  Inputs=+-
  CopyRight2 : Subsystem  Description=|  mask(Copyright Information){none=on}
      | Copyright info block.                                               
      |                                                                     
      | Place copyright information at the top of every subsystem in design.
      mask prompts: none "No parameters"
      mask help: Place copyright information at the top of every subsystem in design.
      mask Display:
      | NxtrConf = 'Nexteer Confidential';
      | 
      | sys = bdroot; %handle for the current model ("system")
      | first = get_param(sys,'Created');
      | if(isempty(first))
      |     first = datestr(now,'yyyy');
      | else
      |     first = first(end-3:end);  %year is last four digits
      | end
      | 
      | last = get_param(sys,'LastModifiedDate');
      | if isempty(last)
      |     last = datestr(now,'yyyy');
      | else
      |     last = last(end-3:end);
      | end
      | 
      | if strcmp(first,last)
      |     fprintf('%s -- Copyright %s Nexteer',NxtrConf,first)
      | else
      |     fprintf('%s -- %s%s- %s Nexteer',NxtrConf,char(169),first,last)
      | end
  D_SQRT3OVR2_ULS2 : Constant  RequirementInfo={'linktype_rmi_doors' '0000bb44 (/E-STEER Core/SubSystem Specifications/Application Functions/SF99/SF105A Current Regulator and Voltage Limiter)' '#SF105A_212' 'true' 'REQ: SF105A_212' '' } %GIDa_7c090ab4_3e11_4a51_864b_1175f8b0fffd  Value=ARCHGLBPRM_2OVERSQRT3_ULS_F32  SampleTime=-1
  D_SQRT3OVR2_ULS3 : Constant  RequirementInfo={'linktype_rmi_doors' '0000bb44 (/E-STEER Core/SubSystem Specifications/Application Functions/SF99/SF105A Current Regulator and Voltage Limiter)' '#SF105A_212' 'true' 'REQ: SF105A_212' '' } %GIDa_855f7143_0fd8_4464_9a72_b0eb16b895bd  Value=ARCHGLBPRM_2OVERSQRT3_ULS_F32  SampleTime=-1
  Demux : Demux  RequirementInfo={'linktype_rmi_doors' '0000bb44 (/E-STEER Core/SubSystem Specifications/Application Functions/SF99/SF105A Current Regulator and Voltage Limiter)' '#SF105A_212' 'true' 'REQ: SF105A_212' '' } %GIDa_b4f041f7_9145_4156_a295_824cd2e3b043  Outputs=2
  If Action Subsystem2 : Subsystem  RequirementInfo="{'linktype_rmi_doors' '0000bb44 (/E-STEER Core/SubSystem Specifications/Application Functions/SF99/SF105A Current Regulator and Voltage Limiter)' '#SF105A_189' 'true' 'REQ:  SF105A_189' '' ; 'linktype_rmi_doors' '0000bb44 (/E-STEER Core/SubSystem Specifications/Application Functions/SF99/SF105A Current Regulator and Voltage Limiter)' '#SF105A_212' 'true' 'REQ: SF105A_212' '' } %GIDa_8d5ce8a5_9637_45ba_905e_f8f3271044d4"  TreatAsAtomicUnit=on
  If Action Subsystem3 : Subsystem  RequirementInfo="{'linktype_rmi_doors' '0000bb44 (/E-STEER Core/SubSystem Specifications/Application Functions/SF99/SF105A Current Regulator and Voltage Limiter)' '#SF105A_189' 'true' 'REQ:  SF105A_189' '' ; 'linktype_rmi_doors' '0000bb44 (/E-STEER Core/SubSystem Specifications/Application Functions/SF99/SF105A Current Regulator and Voltage Limiter)' '#SF105A_212' 'true' 'REQ: SF105A_212' '' } %GIDa_a0457bfa_8f29_4d78_8594_a3a6f5ab5c30"  TreatAsAtomicUnit=on
  If1 : If  RequirementInfo="{'linktype_rmi_doors' '0000bb44 (/E-STEER Core/SubSystem Specifications/Application Functions/SF99/SF105A Current Regulator and Voltage Limiter)' '#SF105A_189' 'true' 'REQ:  SF105A_189' '' ; 'linktype_rmi_doors' '0000bb44 (/E-STEER Core/SubSystem Specifications/Application Functions/SF99/SF105A Current Regulator and Voltage Limiter)' '#SF105A_212' 'true' 'REQ: SF105A_212' '' } %GIDa_11d21400_77c9_4c81_9e0d_6b5ff2527e6c"  IfExpression=u1
  Merge1 : Merge  RequirementInfo="{'linktype_rmi_doors' '0000bb44 (/E-STEER Core/SubSystem Specifications/Application Functions/SF99/SF105A Current Regulator and Voltage Limiter)' '#SF105A_189' 'true' 'REQ:  SF105A_189' '' ; 'linktype_rmi_doors' '0000bb44 (/E-STEER Core/SubSystem Specifications/Application Functions/SF99/SF105A Current Regulator and Voltage Limiter)' '#SF105A_212' 'true' 'REQ: SF105A_212' '' } %GIDa_b4df3d7d_175d_40bc_9596_c41cc84c245a"
  Mux : Mux  RequirementInfo={'linktype_rmi_doors' '0000bb44 (/E-STEER Core/SubSystem Specifications/Application Functions/SF99/SF105A Current Regulator and Voltage Limiter)' '#SF105A_212' 'true' 'REQ: SF105A_212' '' } %GIDa_243bf615_c7b2_4216_bdd3_add82d3b12aa  Inputs=2
  Mux1 : Mux  RequirementInfo={'linktype_rmi_doors' '0000bb44 (/E-STEER Core/SubSystem Specifications/Application Functions/SF99/SF105A Current Regulator and Voltage Limiter)' '#SF105A_212' 'true' 'REQ: SF105A_212' '' } %GIDa_205f7b3f_7aec_48e9_88d2_aa356588941a  Inputs=2
  Product1 : Product  RequirementInfo={'linktype_rmi_doors' '0000bb44 (/E-STEER Core/SubSystem Specifications/Application Functions/SF99/SF105A Current Regulator and Voltage Limiter)' '#SF105A_212' 'true' 'REQ: SF105A_212' '' } %GIDa_3cdfa017_093f_4abc_8efc_06dc67ecb9a1
  Product2 : Product  RequirementInfo={'linktype_rmi_doors' '0000bb44 (/E-STEER Core/SubSystem Specifications/Application Functions/SF99/SF105A Current Regulator and Voltage Limiter)' '#SF105A_212' 'true' 'REQ: SF105A_212' '' } %GIDa_13f05cde_c0a3_4912_9dff_dcd18f41ff4a
  Product3 : Product  RequirementInfo={'linktype_rmi_doors' '0000bb44 (/E-STEER Core/SubSystem Specifications/Application Functions/SF99/SF105A Current Regulator and Voltage Limiter)' '#SF105A_212' 'true' 'REQ: SF105A_212' '' } %GIDa_121e40e7_fd5b_4597_9d9d_1fe045705111
  Product5 : Product  RequirementInfo={'linktype_rmi_doors' '0000bb44 (/E-STEER Core/SubSystem Specifications/Application Functions/SF99/SF105A Current Regulator and Voltage Limiter)' '#SF105A_212' 'true' 'REQ: SF105A_212' '' } %GIDa_704bbb07_6035_479a_a5b8_eda4a9b50684  Inputs=3
  Product6 : Product  RequirementInfo={'linktype_rmi_doors' '0000bb44 (/E-STEER Core/SubSystem Specifications/Application Functions/SF99/SF105A Current Regulator and Voltage Limiter)' '#SF105A_212' 'true' 'REQ: SF105A_212' '' } %GIDa_5e1628ba_abe6_45e2_825d_d74c907ce54d
  Product7 : Product  RequirementInfo={'linktype_rmi_doors' '0000bb44 (/E-STEER Core/SubSystem Specifications/Application Functions/SF99/SF105A Current Regulator and Voltage Limiter)' '#SF105A_212' 'true' 'REQ: SF105A_212' '' } %GIDa_cdc8df85_3b81_411b_bb71_6bc8bf362b85
  Product8 : Product  RequirementInfo={'linktype_rmi_doors' '0000bb44 (/E-STEER Core/SubSystem Specifications/Application Functions/SF99/SF105A Current Regulator and Voltage Limiter)' '#SF105A_212' 'true' 'REQ: SF105A_212' '' } %GIDa_c228cd1e_e56f_44b3_ad02_740fe0f09447  Inputs=3
  Product9 : Product  RequirementInfo={'linktype_rmi_doors' '0000bb44 (/E-STEER Core/SubSystem Specifications/Application Functions/SF99/SF105A Current Regulator and Voltage Limiter)' '#SF105A_212' 'true' 'REQ: SF105A_212' '' } %GIDa_161dcef5_4ab3_4f95_9b0c_c277200ca5f0
  k_MtrVel_Offset1 : Constant  RequirementInfo={'linktype_rmi_doors' '0000bb44 (/E-STEER Core/SubSystem Specifications/Application Functions/SF99/SF105A Current Regulator and Voltage Limiter)' '#SF105A_210' 'true' 'REQ: SF105A_210' '' ; 'linktype_rmi_doors' '0000bb44 (/E-STEER Core/SubSystem Specifications/Application Functions/SF99/SF105A Current Regulator and Voltage Limiter)' '#SF105A_212' 'true' 'REQ: SF105A_212' '' } %GIDa_c0d39cc7_1ec8_4475_8951_f01a845b848b  Value=MotCurrRegVltgLimrMotCurrPredEna  VectorParams1D=off
  k_MtrVel_Offset6 : Constant  RequirementInfo={'linktype_rmi_doors' '0000bb44 (/E-STEER Core/SubSystem Specifications/Application Functions/SF99/SF105A Current Regulator and Voltage Limiter)' '#SF105A_211' 'true' 'REQ: SF105A_211' '' } %GIDa_2082564c_893f_4978_833e_af621bc5420b  Value=MotCurrRegVltgLimrMotCurrPredTi
  MotCurrQaxPred : Outport  RequirementInfo={'linktype_rmi_doors' '0000bb44 (/E-STEER Core/SubSystem Specifications/Application Functions/SF99/SF105A Current Regulator and Voltage Limiter)' '#SF105A_212' 'true' 'REQ: SF105A_212' '' } %GIDa_60fd812a_7082_4417_8ef9_477065148217
  MotCurrDaxPred : Outport  RequirementInfo={'linktype_rmi_doors' '0000bb44 (/E-STEER Core/SubSystem Specifications/Application Functions/SF99/SF105A Current Regulator and Voltage Limiter)' '#SF105A_212' 'true' 'REQ: SF105A_212' '' } %GIDa_45e2d527_2590_49fb_b191_dbec77062c20  Port=2
  wires:
  MotCurrDax/1 -> [MotCurrDax]
  MotCurrQax/1 -> [MotCurrQax]
  MotREstimd/1 -> [MotREstimd]
  Add1/1 -> Product8/1
  Product8/1 -> Add3/2
  [MotCtrlCurrPredTi] -> Product8/3
  MotCtrlMotVltgDax/1 -> Product6/1
  D_SQRT3OVR2_ULS3/1 -> Product6/2
  Product5/1 -> Add2/2
  [MotCurrDax] -> Add3/1
  Add/1 -> Product5/1
  k_MtrVel_Offset6/1 -> [MotCtrlCurrPredTi]
  MotIvsEstLq/1 -> Product5/2
  MotCtrlMotVltgQax/1 -> Add4/1
  [MotCtrlCurrPredTi] -> Product5/3
  [MotCurrDax] -> Product2/2
  [MotCurrQax] -> Product3/1
  [MotREstimd] -> Product3/2
  [MotCurrQax] -> Add2/1
  MotReacncQax/1 -> Product1/1
  [MotCurrQax] -> Product1/2
  [MotCurrDax] -> Product7/1
  [MotREstimd] -> Product7/2
  Product1/1 -> Add1/2
  Product6/1 -> Add1/1
  Product7/1 -> Add1/3
  MotReacncDax/1 -> Product2/1
  MotIvsEstLd/1 -> Product8/2
  If Action Subsystem2/1(Out1) -> Merge1/1
  If Action Subsystem3/1(Out1) -> Merge1/2
  If1/1 -> If Action Subsystem2/Action
  If1/2 -> If Action Subsystem3/Action
  k_MtrVel_Offset1/1 -> If1/1
  Mux/1 -> If Action Subsystem3/1(In1)
  Merge1/1 -> Demux/1
  Demux/1 -> MotCurrQaxPred/1
  Demux/2 -> MotCurrDaxPred/1
  [MotCurrQax] -> Mux1/1
  [MotCurrDax] -> Mux1/2
  Mux1/1 -> If Action Subsystem2/1(In1)
  Add2/1 -> Mux/1
  Add3/1 -> Mux/2
  MotCtrlMotBackEmfVltg/1 -> Add4/2
  Add4/1 -> Product9/1
  D_SQRT3OVR2_ULS2/1 -> Product9/2
  Product9/1 -> Add/1
  Product2/1 -> Add/2
  Product3/1 -> Add/3

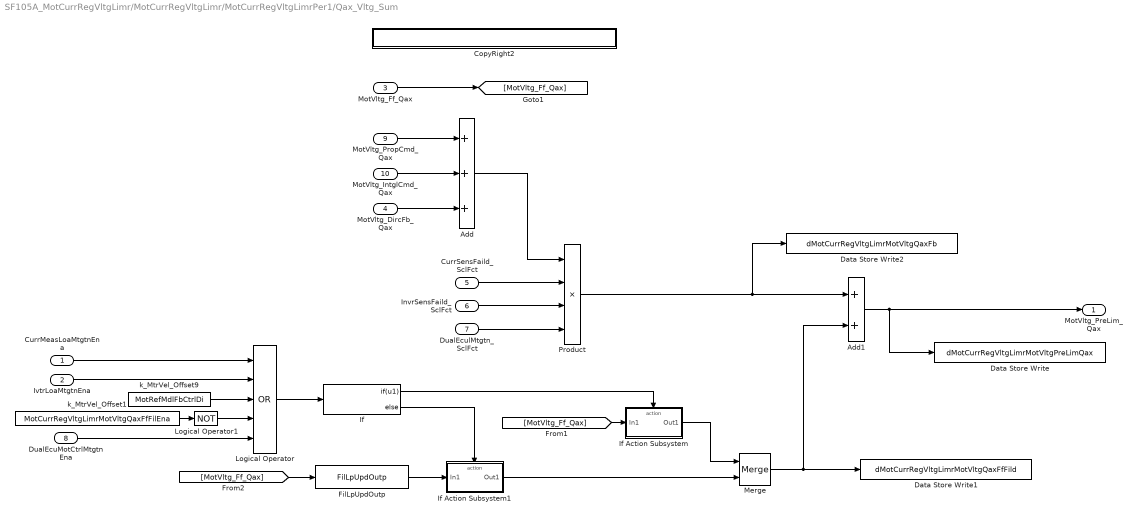
== system SF105A_MotCurrRegVltgLimr/MotCurrRegVltgLimr/MotCurrRegVltgLimrPer1/Qax_Vltg_Sum ==
  CurrMeasLoaMtgtnEna : Inport  RequirementInfo={'linktype_rmi_doors' '0000bb44 (/E-STEER Core/SubSystem Specifications/Application Functions/SF99/SF105A Current Regulator and Voltage Limiter)' '#SF105A_216' 'true' 'REQ: SF105A_216' '' } %GIDa_4ef16ef5_c8b0_4849_a7d6_345e3fb4a3d0
  IvtrLoaMtgtnEna : Inport  RequirementInfo={'linktype_rmi_doors' '0000bb44 (/E-STEER Core/SubSystem Specifications/Application Functions/SF99/SF105A Current Regulator and Voltage Limiter)' '#SF105A_216' 'true' 'REQ: SF105A_216' '' } %GIDa_e6b2f0c6_7f5d_4477_a2d1_387745051d30  Port=2
  MotVltg_Ff_Qax : Inport  RequirementInfo="{'linktype_rmi_doors' '0000bb44 (/E-STEER Core/SubSystem Specifications/Application Functions/SF99/SF105A Current Regulator and Voltage Limiter)' '#SF105A_108' 'true' 'REQ:  SF105A_108' '' } %GIDa_0ef0a3fb_cd34_4518_8fcf_c1f5582b812e"  Port=3
  MotVltg_DircFb_Qax : Inport  RequirementInfo="{'linktype_rmi_doors' '0000bb44 (/E-STEER Core/SubSystem Specifications/Application Functions/SF99/SF105A Current Regulator and Voltage Limiter)' '#SF105A_107' 'true' 'REQ:  SF105A_107' '' } %GIDa_b80b9de4_8ce3_47b3_84b1_11b59751a337"  Port=4
  CurrSensFaild_SclFct : Inport  RequirementInfo="{'linktype_rmi_doors' '0000bb44 (/E-STEER Core/SubSystem Specifications/Application Functions/SF99/SF105A Current Regulator and Voltage Limiter)' '#SF105A_107' 'true' 'REQ:  SF105A_107' '' } %GIDa_46e202e6_4ab9_4636_aba8_00bda1b4f925"  Port=5
  InvrSensFaild_SclFct : Inport  RequirementInfo="{'linktype_rmi_doors' '0000bb44 (/E-STEER Core/SubSystem Specifications/Application Functions/SF99/SF105A Current Regulator and Voltage Limiter)' '#SF105A_107' 'true' 'REQ:  SF105A_107' '' } %GIDa_7cf9fee2_0aec_4102_b7a9_3aae2a97180c"  Port=6
  DualEculMtgtn_SclFct : Inport  RequirementInfo={'linktype_rmi_doors' '0000bb44 (/E-STEER Core/SubSystem Specifications/Application Functions/SF99/SF105A Current Regulator and Voltage Limiter)' '#SF105A_107' 'true' 'REQ: SF105A_107' '' } %GIDa_a3eeb2e9_9e6d_4752_b6aa_ed5e3c20bcf2  Port=7
  DualEcuMotCtrlMtgtnEna : Inport  RequirementInfo={'linktype_rmi_doors' '0000bb44 (/E-STEER Core/SubSystem Specifications/Application Functions/SF99/SF105A Current Regulator and Voltage Limiter)' '#SF105A_216' 'true' 'REQ: SF105A_216' '' } %GIDa_c51a38b2_8783_4885_90fc_c4be2e695783  Port=8
  MotVltg_PropCmd_Qax : Inport  RequirementInfo="{'linktype_rmi_doors' '0000bb44 (/E-STEER Core/SubSystem Specifications/Application Functions/SF99/SF105A Current Regulator and Voltage Limiter)' '#SF105A_107' 'true' 'REQ:  SF105A_107' '' } %GIDa_84f52dab_09ce_4ea8_8626_f5a9154f8b39"  Port=9
  MotVltg_IntglCmd_Qax : Inport  RequirementInfo="{'linktype_rmi_doors' '0000bb44 (/E-STEER Core/SubSystem Specifications/Application Functions/SF99/SF105A Current Regulator and Voltage Limiter)' '#SF105A_107' 'true' 'REQ:  SF105A_107' '' } %GIDa_77690a1e_a127_4045_b256_4d3277884e54"  Port=10
  Add : Sum  RequirementInfo="{'linktype_rmi_doors' '0000bb44 (/E-STEER Core/SubSystem Specifications/Application Functions/SF99/SF105A Current Regulator and Voltage Limiter)' '#SF105A_107' 'true' 'REQ:  SF105A_107' '' } %GIDa_126dcefb_f6a1_43eb_b44d_8e6ba3895d42"  Inputs=+++
  Add1 : Sum  RequirementInfo="{'linktype_rmi_doors' '0000bb44 (/E-STEER Core/SubSystem Specifications/Application Functions/SF99/SF105A Current Regulator and Voltage Limiter)' '#SF105A_108' 'true' 'REQ:  SF105A_108' '' } %GIDa_3de0906f_69b9_4ea3_b963_6d1d25731bb9"
  CopyRight2 : Subsystem  Description=|  mask(Copyright Information){none=on}
      | Copyright info block.                                               
      |                                                                     
      | Place copyright information at the top of every subsystem in design.
      mask prompts: none "No parameters"
      mask help: Place copyright information at the top of every subsystem in design.
      mask Display:
      | NxtrConf = 'Nexteer Confidential';
      | 
      | sys = bdroot; %handle for the current model ("system")
      | first = get_param(sys,'Created');
      | if(isempty(first))
      |     first = datestr(now,'yyyy');
      | else
      |     first = first(end-3:end);  %year is last four digits
      | end
      | 
      | last = get_param(sys,'LastModifiedDate');
      | if isempty(last)
      |     last = datestr(now,'yyyy');
      | else
      |     last = last(end-3:end);
      | end
      | 
      | if strcmp(first,last)
      |     fprintf('%s -- Copyright %s Nexteer',NxtrConf,first)
      | else
      |     fprintf('%s -- %s%s- %s Nexteer',NxtrConf,char(169),first,last)
      | end
  Data Store Write : DataStoreWrite  DataStoreName=dMotCurrRegVltgLimrMotVltgPreLimQax
  Data Store Write1 : DataStoreWrite  DataStoreName=dMotCurrRegVltgLimrMotVltgQaxFfFild
  Data Store Write2 : DataStoreWrite  DataStoreName=dMotCurrRegVltgLimrMotVltgQaxFb
  FilLpUpdOutp : Fil/FilLpUpdOutp  RequirementInfo={'linktype_rmi_doors' '0000bb44 (/E-STEER Core/SubSystem Specifications/Application Functions/SF99/SF105A Current Regulator and Voltage Limiter)' '#SF105A_216' 'true' 'REQ: SF105A_216' '' } %GIDa_d1b5d23d_4bd5_44d2_889f_55b3550a608e  StVar=MotVltgQaxFfLpFil
      settings: AttributesFormatString=StVar: %<StVar>
  If : If  RequirementInfo={'linktype_rmi_doors' '0000bb44 (/E-STEER Core/SubSystem Specifications/Application Functions/SF99/SF105A Current Regulator and Voltage Limiter)' '#SF105A_216' 'true' 'REQ: SF105A_216' '' } %GIDa_deba95ce_b39b_47d1_a8ae_64c4e8c759ee  IfExpression=u1
  If Action Subsystem : Subsystem  RequirementInfo={'linktype_rmi_doors' '0000bb44 (/E-STEER Core/SubSystem Specifications/Application Functions/SF99/SF105A Current Regulator and Voltage Limiter)' '#SF105A_216' 'true' 'REQ: SF105A_216' '' } %GIDa_5c77bbda_ad12_4be3_a744_234d77d7a724  TreatAsAtomicUnit=on
  If Action Subsystem1 : Subsystem  RequirementInfo={'linktype_rmi_doors' '0000bb44 (/E-STEER Core/SubSystem Specifications/Application Functions/SF99/SF105A Current Regulator and Voltage Limiter)' '#SF105A_216' 'true' 'REQ: SF105A_216' '' } %GIDa_79080d8a_ebea_49ae_8611_87746443de90  TreatAsAtomicUnit=on
  Logical Operator : Logic  RequirementInfo={'linktype_rmi_doors' '0000bb44 (/E-STEER Core/SubSystem Specifications/Application Functions/SF99/SF105A Current Regulator and Voltage Limiter)' '#SF105A_216' 'true' 'REQ: SF105A_216' '' } %GIDa_29189a1d_1c98_4094_8931_0e6752d1eaab  Operator=OR  Inputs=5  AllPortsSameDT=off  OutDataTypeStr=boolean
  Logical Operator1 : Logic  RequirementInfo={'linktype_rmi_doors' '0000bb44 (/E-STEER Core/SubSystem Specifications/Application Functions/SF99/SF105A Current Regulator and Voltage Limiter)' '#SF105A_216' 'true' 'REQ: SF105A_216' '' } %GIDa_5fadc188_a838_4860_9d9c_491f614177a1  Operator=NOT  Inputs=4  AllPortsSameDT=off  OutDataTypeStr=boolean
  Merge : Merge  RequirementInfo={'linktype_rmi_doors' '0000bb44 (/E-STEER Core/SubSystem Specifications/Application Functions/SF99/SF105A Current Regulator and Voltage Limiter)' '#SF105A_216' 'true' 'REQ: SF105A_216' '' } %GIDa_d605c909_7874_4afd_a7e3_769c43d403e1
  Product : Product  RequirementInfo="{'linktype_rmi_doors' '0000bb44 (/E-STEER Core/SubSystem Specifications/Application Functions/SF99/SF105A Current Regulator and Voltage Limiter)' '#SF105A_107' 'true' 'REQ:  SF105A_107' '' } %GIDa_135e9b25_6194_4318_a32a_270e305ff0e1"  Inputs=4
  k_MtrVel_Offset1 : Constant  RequirementInfo={'linktype_rmi_doors' '0000bb44 (/E-STEER Core/SubSystem Specifications/Application Functions/SF99/SF105A Current Regulator and Voltage Limiter)' '#SF105A_216' 'true' 'REQ: SF105A_216' '' } %GIDa_96df3536_1b9f_4daf_8c0c_c75607278ad3  Value=MotCurrRegVltgLimrMotVltgQaxFfFilEna
  k_MtrVel_Offset9 : Constant  RequirementInfo={'linktype_rmi_doors' '0000bb44 (/E-STEER Core/SubSystem Specifications/Application Functions/SF99/SF105A Current Regulator and Voltage Limiter)' '#SF105A_216' 'true' 'REQ: SF105A_216' '' } %GIDa_c7679e39_d257_447c_9416_105348c2431e  Value=MotRefMdlFbCtrlDi
  MotVltg_PreLim_Qax : Outport  RequirementInfo="{'linktype_rmi_doors' '0000bb44 (/E-STEER Core/SubSystem Specifications/Application Functions/SF99/SF105A Current Regulator and Voltage Limiter)' '#SF105A_108' 'true' 'REQ:  SF105A_108' '' } %GIDa_e3e967bf_f838_4163_8b54_d961a38b5185"
  wires:
  Add/1 -> Product/1
  InvrSensFaild_SclFct/1 -> Product/3
  CurrSensFaild_SclFct/1 -> Product/2
  Product/1 -> Data Store Write2/1, Add1/1
  MotVltg_Ff_Qax/1 -> [MotVltg_Ff_Qax]
  Add1/1 -> Data Store Write/1, MotVltg_PreLim_Qax/1
  MotVltg_PropCmd_Qax/1 -> Add/1
  MotVltg_IntglCmd_Qax/1 -> Add/2
  MotVltg_DircFb_Qax/1 -> Add/3
  k_MtrVel_Offset1/1 -> Logical Operator1/1
  Logical Operator1/1 -> Logical Operator/4
  k_MtrVel_Offset9/1 -> Logical Operator/3
  IvtrLoaMtgtnEna/1 -> Logical Operator/2
  CurrMeasLoaMtgtnEna/1 -> Logical Operator/1
  Logical Operator/1 -> If/1
  If/2 -> If Action Subsystem1/Action
  If/1 -> If Action Subsystem/Action
  If Action Subsystem/1(Out1) -> Merge/1
  If Action Subsystem1/1(Out1) -> Merge/2
  [MotVltg_Ff_Qax] -> If Action Subsystem/1(In1)
  [MotVltg_Ff_Qax] -> FilLpUpdOutp/1
  FilLpUpdOutp/1 -> If Action Subsystem1/1(In1)
  Merge/1 -> Data Store Write1/1, Add1/2
  DualEcuMotCtrlMtgtnEna/1 -> Logical Operator/5
  DualEculMtgtn_SclFct/1 -> Product/4
